simulink model "manual_control_new"  (R2023a)
settings: Solver=FixedStepAuto  StartTime=0.0  StopTime=inf  FixedStep=Ts_slk  RelTol=1e-3  EnableMultiTasking=on
undefined symbols (not defined in the file): dev, IMU_w_b_bias, Main, meas_pole, P0_phth, P0_ps, pwm_output0, Q_phth, q_ps, R_phth, r_ps, Rz, Ts_EKF_integr, Ts_EKF_meas, Ts_slk, x0_phth, x0_ps
libraries: px4Sensorslib x4, px4lib x1, sharedtransform x1
(part 2 of 2)

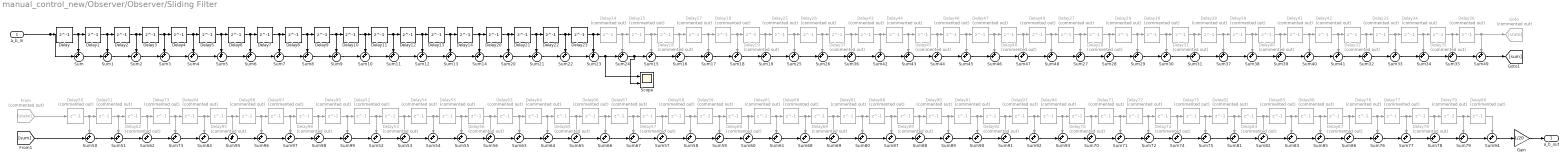
== system manual_control_new/Observer/Observer/Sliding Filter ==
  a_b_in : Inport
  Delay{,1..14,20..23} (19 alike) : Delay  DelayLength=1  SampleTime=Ts_slk
  Delay{15..19,24..99} (81 alike) : Delay  Commented=on  DelayLength=1  SampleTime=Ts_slk
  From : From  Commented=on  GotoTag=state
  Gain : Gain  Gain=1/20
  Goto : Goto  Commented=on  GotoTag=state
  Scope : Scope  NumInputPorts=2
  Sum{,1..99} (100 alike) : Sum  Inputs=++|
  a_b_out : Outport
  wires:
  Delay/1 -> Sum/1, Delay1/1
  Delay1/1 -> Sum1/1, Delay2/1
  Delay2/1 -> Sum2/1, Delay3/1
  Delay3/1 -> Sum3/1, Delay4/1
  Sum/1 -> Sum1/2
  Sum1/1 -> Sum2/2
  Sum2/1 -> Sum3/2
  Sum3/1 -> Sum4/2
  Delay4/1 -> Delay5/1, Sum4/1
  Sum4/1 -> Sum5/2
  a_b_in/1 -> Sum/2, Delay/1
  Delay5/1 -> Sum5/1, Delay6/1
  Delay6/1 -> Sum6/1, Delay7/1
  Sum5/1 -> Sum6/2
  Sum6/1 -> Sum7/2
  Sum7/1 -> Sum8/2
  Delay7/1 -> Sum7/1, Delay8/1
  Delay8/1 -> Delay9/1, Sum8/1
  Delay9/1 -> Sum9/1, Delay10/1
  Delay10/1 -> Sum10/1, Delay11/1
  Delay11/1 -> Sum11/1, Delay12/1
  Delay12/1 -> Sum12/1, Delay13/1
  Delay13/1 -> Sum13/1, Delay14/1
  Sum11/1 -> Sum12/2
  Sum12/1 -> Sum13/2
  Sum13/1 -> Sum14/2
  Sum8/1 -> Sum9/2
  Sum9/1 -> Sum10/2
  Sum10/1 -> Sum11/2
  Delay14/1 -> Delay20/1, Sum14/1
  Delay19/1 -> Delay25/1, Sum19/1
  Sum16/1 -> Sum17/2
  Delay15/1 -> Sum15/1, Delay16/1
  Sum24/1 -> Scope/2, Sum15/2
  Sum17/1 -> Sum18/2
  Delay23/1 -> Delay24/1, Sum23/1
  Delay24/1 -> Sum24/1, Delay15/1
  Sum20/1 -> Sum21/2
  Delay22/1 -> Sum22/1, Delay23/1
  Delay18/1 -> Sum18/1, Delay19/1
  Sum23/1 -> Scope/1, Sum24/2
  Sum22/1 -> Sum23/2
  Sum14/1 -> Sum20/2
  Delay20/1 -> Sum20/1, Delay21/1
  Delay17/1 -> Sum17/1, Delay18/1
  Sum18/1 -> Sum19/2
  Delay21/1 -> Sum21/1, Delay22/1
  Delay16/1 -> Sum16/1, Delay17/1
  Sum15/1 -> Sum16/2
  Sum21/1 -> Sum22/2
  Sum41/1 -> Sum32/2
  Delay32/1 -> Sum32/1, Delay33/1
  Sum33/1 -> Sum34/2
  Delay42/1 -> Sum41/1, Delay32/1
  Sum37/1 -> Sum38/2
  Delay41/1 -> Delay42/1, Sum40/1
  Delay31/1 -> Delay38/1, Sum31/1
  Sum28/1 -> Sum29/2
  Delay28/1 -> Sum28/1, Delay29/1
  Delay27/1 -> Sum27/1, Delay28/1
  Delay49/1 -> Sum48/1, Delay27/1
  Sum48/1 -> Sum27/2
  Sum29/1 -> Sum30/2
  Delay48/1 -> Delay49/1, Sum47/1
  Sum44/1 -> Sum45/2
  Delay47/1 -> Sum46/1, Delay48/1
  Delay45/1 -> Sum44/1, Delay46/1
  Delay39/1 -> Sum38/1, Delay40/1
  Sum47/1 -> Sum48/2
  Delay38/1 -> Sum37/1, Delay39/1
  Sum40/1 -> Sum41/2
  Sum46/1 -> Sum47/2
  Sum34/1 -> Sum35/2
  Delay29/1 -> Sum29/1, Delay30/1
  Sum32/1 -> Sum33/2
  Delay40/1 -> Sum39/1, Delay41/1
  Delay46/1 -> Sum45/1, Delay47/1
  Delay33/1 -> Sum33/1, Delay34/1
  Sum27/1 -> Sum28/2
  Delay30/1 -> Sum30/1, Delay31/1
  Sum36/1 -> Sum42/2
  Delay44/1 -> Delay45/1, Sum43/1
  Sum39/1 -> Sum40/2
  Delay37/1 -> Sum36/1, Delay43/1
  Sum26/1 -> Sum36/2
  Sum43/1 -> Sum44/2
  Sum25/1 -> Sum26/2
  Delay35/1 -> Sum35/1, Delay36/1
  Sum42/1 -> Sum43/2
  Delay43/1 -> Sum42/1, Delay44/1
  Sum30/1 -> Sum31/2
  Sum45/1 -> Sum46/2
  Sum31/1 -> Sum37/2
  Delay26/1 -> Sum26/1, Delay37/1
  Delay25/1 -> Sum25/1, Delay26/1
  Delay34/1 -> Sum34/1, Delay35/1
  Sum38/1 -> Sum39/2
  Sum35/1 -> Sum49/2
  Sum19/1 -> Sum25/2
  Delay36/1 -> Goto/1, Sum49/1
  Sum49/1 -> [sum]
  Delay68/1 -> Sum68/1, Delay69/1
  Sum82/1 -> Sum83/2
  Sum68/1 -> Sum69/2
  Sum75/1 -> Sum81/2
  Delay88/1 -> Sum87/1, Delay89/1
  Delay79/1 -> Sum79/1, Delay80/1
  Sum74/1 -> Sum75/2
  Delay69/1 -> Sum69/1, Delay81/1
  Sum90/1 -> Sum91/2
  Sum83/1 -> Sum85/2
  Sum80/1 -> Sum87/2
  Sum88/1 -> Sum89/2
  Sum69/1 -> Sum80/2
  Sum70/1 -> Sum71/2
  Delay78/1 -> Sum78/1, Delay79/1
  Sum92/1 -> Sum93/2
  Sum78/1 -> Sum79/2
  Sum91/1 -> Sum92/2
  Sum85/1 -> Sum86/2
  Sum76/1 -> Sum77/2
  Delay72/1 -> Sum72/1, Delay74/1
  Delay82/1 -> Sum81/1, Delay83/1
  Sum72/1 -> Sum74/2
  Delay94/1 -> Sum93/1, Delay70/1
  Delay85/1 -> Sum83/1, Delay86/1
  Delay74/1 -> Sum74/1, Delay75/1
  Sum93/1 -> Sum70/2
  Delay90/1 -> Sum89/1, Delay91/1
  Delay92/1 -> Sum91/1, Delay93/1
  Delay93/1 -> Delay94/1, Sum92/1
  Delay75/1 -> Delay82/1, Sum75/1
  Sum71/1 -> Sum72/2
  Delay71/1 -> Sum71/1, Delay72/1
  Delay70/1 -> Sum70/1, Delay71/1
  Sum67/1 -> Sum57/2
  Delay57/1 -> Sum57/1, Delay58/1
  Sum58/1 -> Sum59/2
  Sum89/1 -> Sum90/2
  Delay61/1 -> Delay68/1, Sum61/1
  Delay67/1 -> Sum67/1, Delay57/1
  Sum63/1 -> Sum64/2
  Delay66/1 -> Delay67/1, Sum66/1
  Sum94/1 -> Gain/1
  Sum81/1 -> Sum82/2
  Sum77/1 -> Sum78/2
  Delay87/1 -> Sum86/1, Delay76/1
  Delay76/1 -> Sum76/1, Delay77/1
  Delay86/1 -> Delay87/1, Sum85/1
  Sum86/1 -> Sum76/2
  Sum53/1 -> Sum54/2
  Delay53/1 -> Sum53/1, Delay54/1
  Delay56/1 -> Delay63/1, Sum56/1
  Delay52/1 -> Sum52/1, Delay53/1
  Delay99/1 -> Sum99/1, Delay52/1
  Sum99/1 -> Sum52/2
  Sum54/1 -> Sum55/2
  Delay98/1 -> Delay99/1, Sum98/1
  Sum95/1 -> Sum96/2
  Delay97/1 -> Sum97/1, Delay98/1
  Delay95/1 -> Sum95/1, Delay96/1
  Delay55/1 -> Sum55/1, Delay56/1
  Sum98/1 -> Sum99/2
  Sum64/1 -> Sum65/2
  Delay64/1 -> Sum64/1, Delay65/1
  Delay58/1 -> Sum58/1, Delay59/1
  Delay81/1 -> Sum80/1, Delay88/1
  Delay63/1 -> Sum63/1, Delay64/1
  Sum66/1 -> Sum67/2
  Sum97/1 -> Sum98/2
  Delay77/1 -> Sum77/1, Delay78/1
  Sum59/1 -> Sum60/2
  Delay54/1 -> Sum54/1, Delay55/1
  Sum57/1 -> Sum58/2
  Delay89/1 -> Delay90/1, Sum88/1
  Delay65/1 -> Sum65/1, Delay66/1
  Delay96/1 -> Sum96/1, Delay97/1
  Sum52/1 -> Sum53/2
  From/1 -> Delay50/1
  Delay83/1 -> Sum82/1, Delay85/1
  Sum62/1 -> Sum73/2
  Delay84/1 -> Delay95/1, Sum84/1
  Sum65/1 -> Sum66/2
  Sum87/1 -> Sum88/2
  Delay62/1 -> Sum62/1, Delay73/1
  Sum51/1 -> Sum62/2
  Delay91/1 -> Sum90/1, Delay92/1
  Sum84/1 -> Sum95/2
  Sum50/1 -> Sum51/2
  Delay60/1 -> Sum60/1, Delay61/1
  Sum73/1 -> Sum84/2
  Delay73/1 -> Sum73/1, Delay84/1
  Sum55/1 -> Sum56/2
  Sum61/1 -> Sum68/2
  Delay80/1 -> Sum94/1
  Sum96/1 -> Sum97/2
  Sum79/1 -> Sum94/2
  Sum56/1 -> Sum63/2
  Delay51/1 -> Sum51/1, Delay62/1
  Delay50/1 -> Sum50/1, Delay51/1
  Delay59/1 -> Sum59/1, Delay60/1
  Sum60/1 -> Sum61/2
  Gain/1 -> a_b_out/1
  [sum] -> Sum50/2

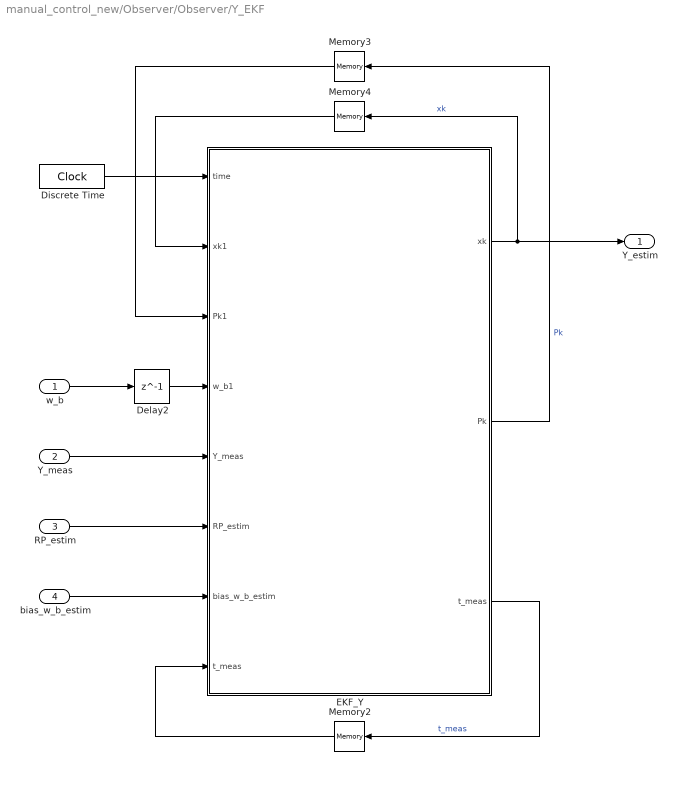
== system manual_control_new/Observer/Observer/Y_EKF ==
  w_b : Inport
  Y_meas : Inport  Port=2
  RP_estim : Inport  Port=3
  bias_w_b_estim : Inport  Port=4
  Delay2 : Delay  DelayLength=1  SampleTime=Ts_EKF_meas
  Discrete Time : DigitalClock  SampleTime=Ts_slk
  EKF_Y : MATLAB Function  TreatAsAtomicUnit=on
  Memory2 : Memory
  Memory3 : Memory  InitialCondition=ones(1,1)*P0_ps
  Memory4 : Memory  InitialCondition=ones(1,1)*x0_ps
  Y_estim : Outport
  wires:
  w_b/1 -> Delay2/1
  EKF_Y/2(Pk) -> Memory3/1  "Pk"
  Memory2/1 -> EKF_Y/8("t_meas ")
  EKF_Y/3(t_meas) -> Memory2/1  "t_meas"
  Y_meas/1 -> EKF_Y/5(Y_meas)
  Discrete Time/1 -> EKF_Y/1(time)
  Memory3/1 -> EKF_Y/3(Pk1)
  Delay2/1 -> EKF_Y/4(w_b1)
  Memory4/1 -> EKF_Y/2(xk1)
  EKF_Y/1(xk) -> Memory4/1, Y_estim/1  "xk"
  bias_w_b_estim/1 -> EKF_Y/7(bias_w_b_estim)
  RP_estim/1 -> EKF_Y/6(RP_estim)

== system manual_control_new/Observer/Subsystem/unlimited RPY1 ==
  RPYin : Inport
  Memory : Memory
  Memory1 : Memory
  unlimited RPY : MATLAB Function  TreatAsAtomicUnit=on
  RPYout : Outport
  wires:
  RPYin/1 -> unlimited RPY/1("RPY ")
  unlimited RPY/1(RPY) -> Memory/1, RPYout/1
  Memory/1 -> unlimited RPY/2(RPY1)
  unlimited RPY/2(init) -> Memory1/1
  Memory1/1 -> unlimited RPY/3("init ")

== system manual_control_new/PX4/U + BIAS/input1 ==
  In1 : Inport
  Constant : Constant  Value=1000  SampleTime=Ts_slk
  Data Type Conversion1 : DataTypeConversion  OutDataTypeStr=uint16  SaturateOnIntegerOverflow=off  RndMeth=Floor
  Sum : Sum  Inputs=|++
  Out1 : Outport
  wires:
  Sum/1 -> Data Type Conversion1/1
  In1/1 -> Sum/1
  Constant/1 -> Sum/2
  Data Type Conversion1/1 -> Out1/1

== system manual_control_new/PX4/U + BIAS/input2 ==
  In1 : Inport
  Constant : Constant  Value=1000  SampleTime=Ts_slk
  Data Type Conversion1 : DataTypeConversion  OutDataTypeStr=uint16  SaturateOnIntegerOverflow=off  RndMeth=Floor
  Sum : Sum  Inputs=|++
  Out1 : Outport
  wires:
  Sum/1 -> Data Type Conversion1/1
  In1/1 -> Sum/1
  Constant/1 -> Sum/2
  Data Type Conversion1/1 -> Out1/1

== system manual_control_new/PX4/U + BIAS/input3 ==
  In1 : Inport
  Constant : Constant  Value=1000  SampleTime=Ts_slk
  Data Type Conversion1 : DataTypeConversion  OutDataTypeStr=uint16  SaturateOnIntegerOverflow=off  RndMeth=Floor
  Sum : Sum  Inputs=|++
  Out1 : Outport
  wires:
  Sum/1 -> Data Type Conversion1/1
  In1/1 -> Sum/1
  Constant/1 -> Sum/2
  Data Type Conversion1/1 -> Out1/1

== system manual_control_new/PX4/U + BIAS/input4 ==
  In1 : Inport
  Constant : Constant  Value=1000  SampleTime=Ts_slk
  Data Type Conversion1 : DataTypeConversion  OutDataTypeStr=uint16  SaturateOnIntegerOverflow=off  RndMeth=Floor
  Sum : Sum  Inputs=|++
  Out1 : Outport
  wires:
  Sum/1 -> Data Type Conversion1/1
  In1/1 -> Sum/1
  Constant/1 -> Sum/2
  Data Type Conversion1/1 -> Out1/1

== matlab function manual_control_new/MATLAB Function3 ==
  data: u input; y1 output; y2 output; y3 output
function [y1,y2,y3] = fcn(u)

y1 = u(1);
y2 = u(2);
y3 = u(3);

== matlab function manual_control_new/Observer/Observer/RP_EKF/MATLAB Function ==
  data: xk input; RP_estim output; bias_w_b_estim output
function [RP_estim, bias_w_b_estim] = state_extraction(xk)

RP_estim        = xk(1:2,1);
bias_w_b_estim  = xk(3:5,1);
end

== matlab function manual_control_new/Observer/MATLAB Function1 ==
  data: u input; y1 output; y2 output; y3 output
function [y1,y2,y3] = fcn(u)

y1 = u(1);
y2 = u(2);
y3 = u(3);

== matlab function manual_control_new/Observer/IMU measurements & rotation/MATLAB Function ==
  data: u input; y output
function y = a_b_roation(u)
y = zeros(3,1);
y(1) = -u(1);
y(2) = +u(2);
y(3) = +u(3);
end

== matlab function manual_control_new/Observer/Observer/RPY_dot_computation ==
  data: time input; w_b input; RPY_estim input; bias_w_b_estim input; Ts_EKF_meas input; RPY_rate1 input; RPY_rate output; t_meas1 input; t_meas1 output
function [RPY_rate,t_meas1] = RPY_dot_computation(time,w_b,RPY_estim,bias_w_b_estim,Ts_EKF_meas,RPY_rate1,t_meas1)

if time - t_meas1 >= Ts_EKF_meas || time == 0
    wp          =       w_b(1,1);               % p-dir of angular velocity w
    wq          =       w_b(2,1);               % q-dir of angular velocity w
    wr          =       w_b(3,1);               % r-dir of angular velocity w

    phi         =       RPY_estim(1,1);         % roll angle (rad)
    theta       =       RPY_estim(2,1);         % pitch angle (rad)
    psi         =       RPY_estim(3,1);         % yaw angle (rad)  
    bias_wp     =       bias_w_b_estim(1,1)*0;    % bias of p-dir of angular velocity w
    bias_wq     =       bias_w_b_estim(2,1)*0;    % bias of q-dir of angular velocity w
    bias_wr     =       bias_w_b_estim(3,1)*0;   % bias of r-dir of angular velocity w

    cph         =       cos(phi);
    cth         =       cos(theta);
    cps         =       cos(psi);
    sph         =       sin(phi);
    sth         =       sin(theta);
    sps         =       sin(psi);
    tth         =       sth/cth;

    % integration step
    t_meas1 = time;
    W_eta = [1,    sph*tth,    cph*tth;
             0,    cph,        -sph;
             0,    sph/cth,    cph/cth;];
    w_b_corrected = [wp-bias_wp; wq-bias_wq; wr-bias_wr;];
    RPY_rate = W_eta*w_b_corrected;
else
    RPY_rate = RPY_rate1;
end
end

== matlab function manual_control_new/Sensors/correct sequence ==
  data: u input; y output
function y  = fcn(u)

y = single([0,0,0]);
y(1) = u(3);
y(2) = u(2);
y(3) = u(1);

== matlab function manual_control_new/Observer/Subsystem/MATLAB Function2 ==
  data: u input; y1 output; y2 output
function [y1,y2] = fcn(u)

y1 = u(1:3);
y2 = u(4:6);
end

== matlab function manual_control_new/Observer/Observer/Median Filter/MATLAB Function ==
  data: u input; y output
function y = fcn(u)
[n,~] = size(u);
n = n/3;
norm = zeros(n,2);
for i = 1:1:n
    u_vect      = u(i*3-2:i*3,1); 
    norm(i,1)   = sqrt(u_vect'*u_vect);     % norm
    norm(i,2)   = i;                        % index
end
for i = 1:n-1
    for j = 1:n-i
        if norm(j,1) > norm(j+1,1)
            % Swap elements
            temp = norm(j,:);
            norm(j,:) = norm(j+1,:);
            norm(j+1,:) = temp;
        end
    end
end
indexMedian = floor(n/2-1);
median = norm(indexMedian,2);
y = u(median*3-2:median*3);
end

== matlab function manual_control_new/Observer/unlimited RPY/unlimited RPY ==
  data: RPY input; RPY output; RPY1 input; init output; init input
function [RPY,init] = unlimited_RPY(RPY,RPY1, init)
if init == 0
    init = 1;
    RPY1 = RPY;
end

for i =1:1:3
    while abs(RPY(i) - RPY1(i)) > pi/2
        RPY(i) = RPY(i) + sign(RPY1(i))*pi;
    end
end
end

== matlab function manual_control_new/Observer/Subsystem/MATLAB Function7 ==
  data: u input; y1 output; y2 output; y3 output
function [y1,y2,y3] = fcn(u)

y1 = u(1);
y2 = u(2);
y3 = u(3);

== matlab function manual_control_new/unlimited RPY2/unlimited RPY ==
  data: RPY input; RPY output; RPY1 input; init output; init input
function [RPY,init] = unlimited_RPY(RPY,RPY1, init)
if init == 0
    init = 1;
    RPY1 = RPY;
end

for i =1:1:3
    while abs(RPY(i) - RPY1(i)) > pi/2
        RPY(i) = RPY(i) + sign(RPY1(i))*pi;
    end
end
end

== matlab function manual_control_new/Observer/Subsystem/unlimited RPY1/unlimited RPY ==
  data: RPY input; RPY output; RPY1 input; init output; init input
function [RPY,init] = unlimited_RPY(RPY,RPY1, init)
if init == 0
    init = 1;
    RPY1 = RPY;
end

for i =1:1:3
    while abs(RPY(i) - RPY1(i)) > pi/2
        RPY(i) = RPY(i) + sign(RPY1(i))*pi;
    end
end
end

== matlab function manual_control_new/Observer/Subsystem/MATLAB Function1 ==
  data: u input; y1 output; y2 output; y3 output
function [y1,y2,y3] = fcn(u)

y1 = u(1);
y2 = u(2);
y3 = u(3);

== matlab function manual_control_new/Observer/IMU measurements & rotation/MATLAB Function1 ==
  data: u input; y output
function y = w_b_roation(u)
y = zeros(3,1);
y(1) = +u(1);
y(2) = -u(2);
y(3) = -u(3);
end

== matlab function manual_control_new/Observer/Observer/Y_computation ==
  data: mf_b input; RP_estim input; Y_meas output
function Y_meas    = Y_computation(mf_b,RP_estim)
% description:
% - a_b             = measured linear acceleration in body-frame
% - w_b             = measured angular velocity in body-frame
% - mf_b            = measured magnetic field in body-frame
% - mf              = measured magnetic field in body-inertia
% - a_b_disturbe    = linear velocity measurement-noise
% - w_b_disturbe    = angular velocity measurement-noise
% - mf_b_disturbe   = magnetic field measurement-noise

% -------------------------------------------------------------------------------------------
% observation: the following computation works only if the angles
% phi,theta,psy are withing angles (-pi/2,+pi/2) (this is an open set, pi/2 is excluded)
% -------------------------------------------------------------------------------------------

ph_estim = RP_estim(1,1);
th_estim = RP_estim(2,1);

sph = sin(ph_estim);
cph = cos(ph_estim);

sth = sin(th_estim);
cth = cos(th_estim);

ps_meas_num   = mf_b(3)*sph - mf_b(2)*cph;
ps_meas_den = mf_b(1)*cth + mf_b(2)*sth*sph + mf_b(3)*sth*cph;
ps_meas = atan2(ps_meas_num, ps_meas_den);

if ps_meas < 0
    ps_meas = ps_meas + 2*pi;
end

Y_meas = ps_meas;
end

== matlab function manual_control_new/Observer/Observer/Y_EKF/EKF_Y ==
  data: time input; xk1 input size=[1,1]; Pk1 input size=[1,1]; w_b1 input; Y_meas input; RP_estim input; bias_w_b_estim input; t_meas input; q_ps parameter; xk output size=[1,1]; Pk output; t_meas output; r_ps parameter; Ts_EKF_integr parameter; Ts_EKF_meas parameter
function [xk,Pk,t_meas] = EKF_Y(time,xk1,Pk1,w_b1,Y_meas,RP_estim,bias_w_b_estim,t_meas,q_ps,r_ps,Ts_EKF_integr,Ts_EKF_meas)

if time - t_meas >= Ts_EKF_meas
    t_meas = time;
    Q = q_ps;
    R = r_ps;

  % INTEGRATION STEP
    % initial condition
    xt1         =       xk1;                        % initial condition for the state
    Pt1         =       Pk1;                        % initial condition for matrix P

    wp1         =       w_b1(1,1);                  % past value of the p-dir of angular velocity w
    wq1         =       w_b1(2,1);                  % past value of the q-dir of angular velocity w
    wr1         =       w_b1(3,1);                  % past value of the r-dir of angular velocity w

    phi         =       RP_estim(1,1);              % estimate of roll angle (rad)
    theta       =       RP_estim(2,1);              % estimate of pitch angle (rad)  

    bias_wp     =       bias_w_b_estim(1,1);        % estimate of bias of p-dir of angular velocity w
    bias_wq     =       bias_w_b_estim(2,1);        % estimate of bias of q-dir of angular velocity w
    bias_wr     =       bias_w_b_estim(3,1);        % estimate of bias of r-dir of angular velocity w
    % integration loop
    Nstep       = floor(Ts_EKF_meas/Ts_EKF_integr); % number of integration steps to performe in the t_meas time windows
    xt          = zeros(1,1);
    Pt          = zeros(1,1);
    for i = 1:1:Nstep
        % state extraction
            psi         =       xt1(1,1);           % roll angle (rad)
        
            cph         =       cos(phi);
            cth         =       cos(theta);
            cps         =       cos(psi);
            sph         =       sin(phi);
            sth         =       sin(theta);
            sps         =       sin(psi);
            tth         =       sth/cth;
        % integration
            Mf = [0,    sph/cth,    cph/cth,    0,  0,  0;];
            Z1 = [wp1-bias_wp; wq1-bias_wq; wr1-bias_wr; bias_wp; bias_wq; bias_wr;];
            f = Mf*Z1;
            xt = xt1 + Ts_EKF_integr*f;
        
            At1 = 0;
            Pt = Pt1 + Ts_EKF_integr*(At1*Pt1 + Pt1*At1' + Q);
        % house keeping
            xt1 = xt;
            Pt1 = Pt;
    end
  % MEASUREMENT STEP
    Ck = [eye(1)];
    Lk = Pt*Ck'/(Ck*Pt*Ck' + R);
    xk = xt + Lk*(Y_meas - Ck*xt);
    Pk = (eye(1) - Lk*Ck)*Pt;
else
    xk = xk1;
    Pk = Pk1;
end
end

== matlab function manual_control_new/Observer/Observer/RP_computation ==
  data: a_b input; RP_meas output
function RP_meas    = RP_computation(a_b)
% description:
% - a_b             = measured linear acceleration in body-frame
% - w_b             = measured angular velocity in body-frame
% - mf_b            = measured magnetic field in body-frame
% - mf              = measured magnetic field in body-inertia
% - a_b_disturbe    = linear velocity measurement-noise
% - w_b_disturbe    = angular velocity measurement-noise
% - mf_b_disturbe   = magnetic field measurement-noise

% -------------------------------------------------------------------------------------------
% observation: the following computation works only if the angles
% phi,theta,psy are withing angles (-pi/2,+pi/2) (this is an open set, pi/2 is excluded)
% -------------------------------------------------------------------------------------------

a_b = -1*a_b;       % need to adjust the sign to use atan2() function correctly

% phi computation
ph_meas = atan2(a_b(2), a_b(3));
sph = sin(ph_meas);
cph = cos(ph_meas);

% theta computation
th_meas = atan2(-a_b(1), (a_b(2)*sph + a_b(3)*cph));

RP_meas = [ph_meas;th_meas];

== matlab function manual_control_new/Observer/Observer/RP_EKF/EKF_RP ==
  data: time input; xk1 input; Pk1 input; w_b1 input; RP_meas input; t_meas input; Q_phth parameter; xk output; Pk output; t_meas output; R_phth parameter; Ts_EKF_integr parameter; Ts_EKF_meas parameter
function [xk,Pk,t_meas] = EKF_RP(time,xk1,Pk1,w_b1,RP_meas,t_meas,Q_phth,R_phth,Ts_EKF_integr,Ts_EKF_meas)

if time - t_meas >= Ts_EKF_meas
    t_meas = time;
    Q = Q_phth;
    R = R_phth;

  % INTEGRATION STEP
    % initial condition
    xt1         =       xk1;                        % initial condition for the state
    Pt1         =       Pk1;                        % initial condition for matrix P
    wp1         =       w_b1(1,1);                  % past value of the p-dir of angular velocity w
    wq1         =       w_b1(2,1);                  % past value of the q-dir of angular velocity w
    wr1         =       w_b1(3,1);                  % past value of the r-dir of angular velocity w
    % integration loop
    Nstep       = floor(Ts_EKF_meas/Ts_EKF_integr); % number of integration steps to performe in the t_meas time windows
    xt          = zeros(5,1);
    Pt          = zeros(5,5);
    for i = 1:1:Nstep
        % state extraction
            phi         =       xt1(1,1);           % roll angle (rad)
            theta       =       xt1(2,1);           % pitch angle (rad)  
            bias_wp     =       xt1(3,1);           % bias of p-dir of angular velocity w
            bias_wq     =       xt1(4,1);           % bias of q-dir of angular velocity w
            bias_wr     =       xt1(5,1);           % bias of r-dir of angular velocity w
        
            cph         =       cos(phi);
            cth         =       cos(theta);
            sph         =       sin(phi);
            sth         =       sin(theta);
            tth         =       sth/cth;
        % integration
            Mf = [1,    sph*tth,    cph*tth,    0,  0,  0;
                  0,    cph,        -sph,       0,  0,  0;
                  0,    0,          0,          0,  0,  0;
                  0,    0,          0,          0,  0,  0;
                  0,    0,          0,          0,  0,  0;];
            Z1 = [wp1-bias_wp; wq1-bias_wq; wr1-bias_wr; bias_wp; bias_wq; bias_wr;];
            f = Mf*Z1;
            xt = xt1 + Ts_EKF_integr*f;
        
            A1 = [cph*tth*(wq1-bias_wq)-sph*tth*(wr1-bias_wr),(sph*(wq1-bias_wq)+cph*(wr1-bias_wr))/cth^2,  -1, -sph*tth,   -cph*tth;];
            A2 = [-sph*(wq1-bias_wq)-cph*(wr1-bias_wr),  0,  0,  -cph,   sph;];
            A3 = [0,  0,  0,  0,  0;];
            A4 = [0,  0,  0,  0,  0;];
            A5 = [0,  0,  0,  0,  0;];
            At1 = [A1; A2; A3; A4; A5;];
            Pt = Pt1 + Ts_EKF_integr*(At1*Pt1 + Pt1*At1' + Q);
        % house keeping
            xt1 = xt;
            Pt1 = Pt;
    end
  % MEASUREMENT STEP
    Ck = [eye(2),zeros(2,3)];
    Lk = Pt*Ck'/(Ck*Pt*Ck' + R);
    xk = xt + Lk*(RP_meas - Ck*xt);
    Pk = (eye(5) - Lk*Ck)*Pt;
else
    xk = xk1;
    Pk = Pk1;
end
end

== matlab function manual_control_new/PX4/Acquisition/MATLAB Function ==
  data: u input; y1 output; y2 output; y3 output; y4 output; y5 output; y6 output
function [y1,y2,y3,y4,y5,y6] = fcn(u)

y1 = u(1);
y2 = u(2);
y3 = u(3);
y4 = u(4);
y5 = u(5);
y6 = u(6);
